simulink model "EVX_Lap_Simulation"  (R2018b)
settings: Solver=FixedStepAuto  StartTime=0  StopTime=100  FixedStep=0.01  MinStep=0.001  RelTol=1e-3
undefined symbols (not defined in the file): Car, dist, DOD, initial_velocity, motorefficiency, motormaxtorque, motorspeedradps, R0model, theta_d, Track_Dist, velocity_dnew, VoltageDOD, x, y
libraries: simulink x4
(part 2 of 3)

== system EVX_Lap_Simulation/EVX Vehicle Model/Powertrain/Brakes ==
  %_Pedal : Inport
  Constant : Constant  Value=2
  Divide : Product  Inputs=*/
  Divide1 : Product  Inputs=*/
  Front Brake Force : Gain  Gain=3000
  Rear Brake Force : Gain  Gain=1500
  Saturation : Saturate  UpperLimit=0  LowerLimit=-1000000
  Wheel Radius Rr : Gain  Gain=0.2
  Wheel radius Fr : Gain  Gain=0.2
  Rear Left Brake : Outport
  Front Left Brake : Outport  Port=2
  Front Right Brake : Outport  Port=3
  Rear Right Brake : Outport  Port=4
  tag scope: T_BrakeFront=global, T_BrakeRear=global
  wires:
  %_Pedal/1 -> Saturation/1
  Rear Brake Force/1 -> Wheel Radius Rr/1
  Front Brake Force/1 -> Wheel radius Fr/1
  Wheel Radius Rr/1 -> Divide1/1, [T_BrakeRear]
  Wheel radius Fr/1 -> Divide/1, [T_BrakeFront]
  Constant/1 -> Divide1/2, Divide/2
  Divide1/1 -> Rear Right Brake/1, Rear Left Brake/1
  Divide/1 -> Front Right Brake/1, Front Left Brake/1
  Saturation/1 -> Rear Brake Force/1, Front Brake Force/1

== system EVX_Lap_Simulation/EVX Vehicle Model/Powertrain/Motor Configuration ==
  %_Pedal : Inport
  radps_Motor1 : Inport  Port=2
  radps_Motor2 : Inport  Port=3
  radps_Motor3 : Inport  Port=4
  radps_Motor4 : Inport  Port=5
  Four Motors : Subsystem  VariantControl=FourMotor
  One Motor : Subsystem  VariantControl=OneMotor
  Two Motors : Subsystem  VariantControl=TwoMotor
  T_FL : Outport
  T_FR : Outport  Port=2
  T_RL : Outport  Port=3
  T_RR : Outport  Port=4
  P_Motor : Outport  Port=5

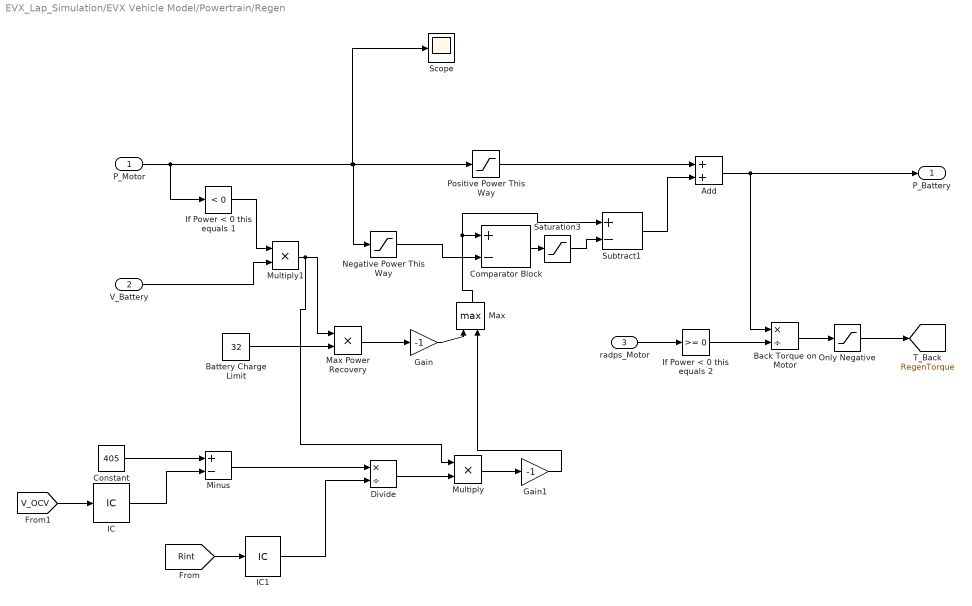
== system EVX_Lap_Simulation/EVX Vehicle Model/Powertrain/Regen ==
  P_Motor : Inport
  V_Battery : Inport  Port=2
  radps_Motor : Inport  Port=3
  Add : Sum
  Back Torque on Motor : Product  Inputs=*/
  Battery Charge Limit : Constant  Value=32
  Comparator Block : Sum  Inputs=+-
  Constant : Constant  Value=405
  Divide : Product  Inputs=*/
  Gain : Gain  Gain=-1
  Gain1 : Gain  Gain=-1
  IC : InitialCondition  Value=400
  IC1 : InitialCondition  Value=0.02
  If Power < 0 this equals 1 : simulink/Logic and Bit Operations/Compare To Zero  relop=<  OutDataTypeStr=boolean
  If Power < 0 this equals 2 : simulink/Logic and Bit Operations/Compare To Zero  relop=>=  OutDataTypeStr=boolean
  Max : MinMax  Function=max  Inputs=2
  Max Power Recovery : Product
  Minus : Sum  Inputs=+-
  Multiply : Product
  Multiply1 : Product
  Negative Power This Way : Saturate  UpperLimit=0  LowerLimit=-10000000
  Only Negative : Saturate  UpperLimit=0  LowerLimit=-10000
  Positive Power This Way : Saturate  UpperLimit=100000  LowerLimit=0
  Saturation3 : Saturate  UpperLimit=0  LowerLimit=-100000
  Scope : Scope
  Subtract1 : Sum  Inputs=+-
  P_Battery : Outport
  tag scope: RegenTorque=global
  wires:
  P_Motor/1 -> Scope/1, Negative Power This Way/1, Positive Power This Way/1, If Power < 0 this equals 1/1
  Positive Power This Way/1 -> Add/1
  Add/1 -> P_Battery/1, Back Torque on Motor/1
  V_Battery/1 -> Multiply1/2
  If Power < 0 this equals 1/1 -> Multiply1/1
  Max Power Recovery/1 -> Gain/1
  radps_Motor/1 -> If Power < 0 this equals 2/1
  Back Torque on Motor/1 -> Only Negative/1
  Only Negative/1 -> [RegenTorque]
  Battery Charge Limit/1 -> Max Power Recovery/2
  Multiply1/1 -> Multiply/1, Max Power Recovery/1
  Negative Power This Way/1 -> Comparator Block/2
  Comparator Block/1 -> Saturation3/1
  Saturation3/1 -> Subtract1/2
  Subtract1/1 -> Add/2
  Minus/1 -> Divide/1
  Constant/1 -> Minus/1
  [V_OCV] -> IC/1
  Divide/1 -> Multiply/2
  Multiply/1 -> Gain1/1
  Gain/1 -> Max/1
  Gain1/1 -> Max/2
  Max/1 -> Subtract1/1, Comparator Block/1
  IC/1 -> Minus/2
  IC1/1 -> Divide/2
  [Rint] -> IC1/1
  If Power < 0 this equals 2/1 -> Back Torque on Motor/2

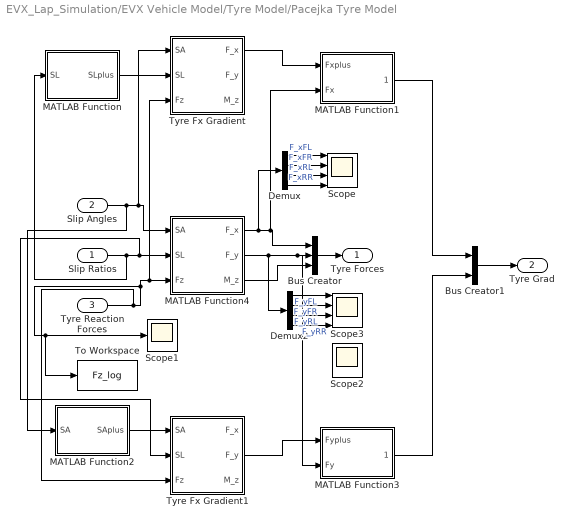
== system EVX_Lap_Simulation/EVX Vehicle Model/Tyre Model/Pacejka Tyre Model ==
  Slip Ratios : Inport
  Slip Angles : Inport  Port=2
  Tyre Reaction Forces : Inport  Port=3
  Bus Creator : BusCreator  Inputs=3
  Bus Creator1 : BusCreator  Inputs=2
  Demux : Demux
  Demux2 : Demux
  MATLAB Function : MATLAB Function  TreatAsAtomicUnit=on
  MATLAB Function1 : MATLAB Function  TreatAsAtomicUnit=on
  MATLAB Function2 : MATLAB Function  TreatAsAtomicUnit=on
  MATLAB Function3 : MATLAB Function  TreatAsAtomicUnit=on
  MATLAB Function4 : MATLAB Function  TreatAsAtomicUnit=on
  Scope : Scope  NumInputPorts=4
  Scope1 : Scope
  Scope2 : Scope  NumInputPorts=4
  Scope3 : Scope  NumInputPorts=4
  To Workspace : ToWorkspace  VariableName=Fz_log  SaveFormat=Timeseries  SampleTime=-1
  Tyre Fx Gradient : MATLAB Function  TreatAsAtomicUnit=on
  Tyre Fx Gradient1 : MATLAB Function  TreatAsAtomicUnit=on
  Tyre Forces : Outport
  Tyre Grad : Outport  Port=2
  wires:
  Bus Creator/1 -> Tyre Forces/1
  Slip Ratios/1 -> MATLAB Function/1(SL), Tyre Fx Gradient1/2(SL), MATLAB Function4/2(SL)
  Slip Angles/1 -> MATLAB Function2/1(SA), Tyre Fx Gradient/1(SA), MATLAB Function4/1(SA)
  Tyre Reaction Forces/1 -> Tyre Fx Gradient1/3(Fz), To Workspace/1, Scope1/1, Tyre Fx Gradient/3(Fz), MATLAB Function4/3(Fz)
  MATLAB Function4/1(F_x) -> Demux/1, MATLAB Function1/2(Fx), Bus Creator/1
  MATLAB Function4/2(F_y) -> Demux2/1, MATLAB Function3/2(Fy), Bus Creator/2
  MATLAB Function4/3(M_z) -> Bus Creator/3
  Demux/1 -> Scope/1  "F_xFL"
  Demux/2 -> Scope/2  "F_xFR"
  Demux/3 -> Scope/3  "F_xRL"
  Demux/4 -> Scope/4  "F_xRR"
  Demux2/1 -> Scope3/1  "F_yFL"
  Demux2/2 -> Scope3/2  "F_yFR"
  Demux2/3 -> Scope3/3  "F_yRL"
  Demux2/4 -> Scope3/4  "F_yRR"
  MATLAB Function/1(SLplus) -> Tyre Fx Gradient/2(SL)
  Tyre Fx Gradient/1(F_x) -> MATLAB Function1/1(Fxplus)
  MATLAB Function2/1(SAplus) -> Tyre Fx Gradient1/1(SA)
  Tyre Fx Gradient1/2(F_y) -> MATLAB Function3/1(Fyplus)
  MATLAB Function1/1(FxGrad) -> Bus Creator1/1
  MATLAB Function3/1(FyGrad) -> Bus Creator1/2
  Bus Creator1/1 -> Tyre Grad/1

== system EVX_Lap_Simulation/EVX Vehicle Model/Vertical Dynamics/Signal Sorting ==
  Signals : Inport
  Bus Creator : BusCreator  Inputs=8
  Bus Creator1 : BusCreator  Inputs=8
  Bus Creator2 : BusCreator  Inputs=8
  Bus Creator3 : BusCreator  Inputs=4
  Bus Creator4 : BusCreator  Inputs=4
  Bus Selector : BusSelector  OutputSignals=A,V,D,Tyre Reaction Forces
  Demux : Demux  Outputs=8
  Demux1 : Demux  Outputs=8
  Demux2 : Demux  Outputs=8
  Demux3 : Demux
  Gain{,1..8} (9 alike) : Gain  Gain=180/pi()
  Named Signals : Outport
  wires:
  Signals/1 -> Bus Selector/1
  Demux/2 -> Bus Creator/2  "Front Right (m)"
  Demux/3 -> Bus Creator/3  "Rear Left (m)"
  Demux/1 -> Bus Creator/1  "Front Left (m)"
  Demux/4 -> Bus Creator/4  "Rear Right (m)"
  Demux/5 -> Bus Creator/5  "Chassis z (m)"
  Demux/6 -> Gain/1  "Pitch (rad)"
  Demux/7 -> Gain1/1  "Front Roll (rad)"
  Demux/8 -> Gain2/1  "Rear Roll (rad)"
  Gain/1 -> Bus Creator/6  "Pitch (deg)"
  Gain2/1 -> Bus Creator/8  "Rear Roll (deg)"
  Gain1/1 -> Bus Creator/7  "Front Roll (deg)"
  Demux1/3 -> Bus Creator1/3  "Rear Left (m/s)"
  Demux1/2 -> Bus Creator1/2  "Front Right (m/s)"
  Gain4/1 -> Bus Creator1/7  "Front Roll (deg/s)"
  Gain5/1 -> Bus Creator1/8  "Rear Roll (deg/s)"
  Demux1/5 -> Bus Creator1/5  "Chassis z (m/s)"
  Demux1/6 -> Gain3/1  "Pitch (rad/s)"
  Demux1/1 -> Bus Creator1/1  "Front Left (m/s)"
  Demux1/8 -> Gain5/1  "Rear Roll (rad/s)"
  Demux1/4 -> Bus Creator1/4  "Rear Right (m/s)"
  Gain3/1 -> Bus Creator1/6  "Pitch (deg/s)"
  Demux1/7 -> Gain4/1  "Front Roll (rad/s)"
  Demux2/4 -> Bus Creator2/4  "Rear Right (m/s^2)"
  Demux2/6 -> Gain6/1  "Pitch (rad/s^2)"
  Demux2/2 -> Bus Creator2/2  "Front Right (m/s^2)"
  Demux2/8 -> Gain8/1  "Rear Roll (rad/s^2)"
  Demux2/1 -> Bus Creator2/1  "Front Left (m/s^2)"
  Demux2/5 -> Bus Creator2/5  "Chassis z (m/s^2)"
  Gain8/1 -> Bus Creator2/8  "Rear Roll (deg/s^2)"
  Gain7/1 -> Bus Creator2/7  "Front Roll (deg/s^2)"
  Demux2/7 -> Gain7/1  "Front Roll (rad/s^2)"
  Demux2/3 -> Bus Creator2/3  "Rear Left (m/s^2)"
  Gain6/1 -> Bus Creator2/6  "Pitch (deg/s^2)"
  Bus Selector/2 -> Demux1/1  "<V>"
  Bus Selector/4 -> Demux3/1  "<Tyre Reaction Forces>"
  Demux3/3 -> Bus Creator3/3  "Rear Left (N)"
  Demux3/4 -> Bus Creator3/4  "Rear Right (N)"
  Demux3/2 -> Bus Creator3/2  "Front Right (N)"
  Demux3/1 -> Bus Creator3/1  "Front Left (N)"
  Bus Creator3/1 -> Bus Creator4/4  "Tyre Forces"
  Bus Creator1/1 -> Bus Creator4/2  "Velocities"
  Bus Creator4/1 -> Named Signals/1  "Vertical Dynamics"
  Bus Selector/1 -> Demux2/1  "<A>"
  Bus Creator/1 -> Bus Creator4/3  "Displacements"
  Bus Selector/3 -> Demux/1  "<D>"
  Bus Creator2/1 -> Bus Creator4/1  "Accelerations"

== system EVX_Lap_Simulation/EVX Vehicle Model/Horizontal Dynamics/Local Dynamics/Subsystem ==
  Signals : Inport
  Bus Creator{,1..3} (4 alike) : BusCreator  Inputs=3
  Bus Selector : BusSelector  OutputSignals=Accelerations,Velocities,Displacements
  Bus Selector1 : BusSelector  OutputSignals=a_x,a_y,ddtheta_z
  Bus Selector2 : BusSelector  OutputSignals=v_x,v_y,dtheta_z
  Bus Selector3 : BusSelector  OutputSignals=d_x,d_y,theta_z
  Named Signals : Outport
  wires:
  Signals/1 -> Bus Selector/1
  Bus Selector/1 -> Bus Selector1/1  "<Accelerations>"
  Bus Selector/2 -> Bus Selector2/1  "<Velocities>"
  Bus Selector/3 -> Bus Selector3/1  "<Displacements>"
  Bus Selector1/1 -> Bus Creator/1  "<a_x>"
  Bus Selector1/2 -> Bus Creator/2  "<a_y>"
  Bus Selector1/3 -> Bus Creator/3  "<ddtheta_z>"
  Bus Selector2/1 -> Bus Creator2/1  "<v_x>"
  Bus Selector2/2 -> Bus Creator2/2  "<v_y>"
  Bus Selector2/3 -> Bus Creator2/3  "<dtheta_z>"
  Bus Selector3/2 -> Bus Creator1/2  "<d_y>"
  Bus Selector3/1 -> Bus Creator1/1  "<d_x>"
  Bus Selector3/3 -> Bus Creator1/3  "<theta_z>"
  Bus Creator2/1 -> Bus Creator3/2  "Velocities"
  Bus Creator/1 -> Bus Creator3/1  "Accelerations"
  Bus Creator1/1 -> Bus Creator3/3  "Displacements"
  Bus Creator3/1 -> Named Signals/1  "Horizontal Dynamics"

== system EVX_Lap_Simulation/EVX Vehicle Model/Powertrain/Battery/Energy ==
  P_Battery : Inport
  Battery Capacity (J) : Constant  Value=25200000
  Battery Percentage : Scope
  Divide : Product  Inputs=/*
  Energy Consumed (J) : Scope
  Energy Remaining (J) : Scope
  Gain : Gain  Gain=100
  Integrator : Integrator
  Minus : Sum  Inputs=+-
  tag scope: E_Battery=global, E_Used=global
  wires:
  Battery Capacity (J)/1 -> Divide/1, Minus/1
  Minus/1 -> Divide/2, [E_Battery], Energy Remaining (J)/1
  Integrator/1 -> Minus/2, [E_Used], Energy Consumed (J)/1
  P_Battery/1 -> Integrator/1
  Divide/1 -> Gain/1
  Gain/1 -> Battery Percentage/1

== system EVX_Lap_Simulation/EVX Vehicle Model/Powertrain/Battery/Heat Generation and Cooling ==
  I_Battery : Inport
  v_Car : Inport  Port=2
  Heat Dissipation (W) : Scope
  Heat Energy (J) : Scope
  Integrator : Integrator
  Internal Resisiatnce : Subsystem
  Multiply : Product
  Square : Math  Operator=square  SaturateOnIntegerOverflow=on
  Temperature and Cooling : Subsystem
  tag scope: E_BatteryHeat=global, P_BatteryHeat=global
  wires:
  Multiply/1 -> [P_BatteryHeat], Temperature and Cooling/1(Heat Generation), Heat Dissipation (W)/1, Integrator/1
  Square/1 -> Multiply/2
  I_Battery/1 -> Square/1
  Integrator/1 -> [E_BatteryHeat], Heat Energy (J)/1
  Internal Resisiatnce/1(R0) -> Multiply/1
  [I_cell] -> Internal Resisiatnce/2(I_cell)
  [SOC_Battery] -> Internal Resisiatnce/1(SOC_Battery)
  v_Car/1 -> Temperature and Cooling/2(v_Car)
  Temperature and Cooling/1(T_Battery) -> Internal Resisiatnce/3(T_Battery)

== system EVX_Lap_Simulation/EVX Vehicle Model/Powertrain/Battery/SOAP ==
  Vocv : Inport
  Divide : Product  Inputs=*/
  Divide2 : Product  Inputs=*/
  Multiply2 : Product
  Scope : Scope
  Subtract1 : Sum  Inputs=+-
  Vcut-off : Constant  Value=242
  tag scope: SOAP_Battery=global, SOAP_ratio=global
  wires:
  Vcut-off/1 -> Subtract1/2
  [Rint] -> Divide2/2
  Subtract1/1 -> Divide2/1
  Divide2/1 -> Multiply2/1
  [V_Battery] -> Multiply2/2
  Multiply2/1 -> Divide/1, Scope/1, [SOAP_Battery]
  Vocv/1 -> Subtract1/1
  [P_Battery] -> Divide/2
  Divide/1 -> [SOAP_ratio]

== system EVX_Lap_Simulation/EVX Vehicle Model/Powertrain/Battery/SOC ==
  Q_Battery : Inport
  %_SOC : Scope
  100% SOC : Constant  Value=72000  VectorParams1D=off
  Battery Charge (As) : Scope
  Divide1 : Product  Inputs=*/
  Gain : Gain  Gain=100
  Minus1 : Sum  Inputs=+-
  SOC_Battery : Outport
  tag scope: SOC_Battery=global
  wires:
  Gain/1 -> [SOC_Battery], SOC_Battery/1, %_SOC/1
  Divide1/1 -> Gain/1
  Minus1/1 -> Battery Charge (As)/1, Divide1/1
  100% SOC/1 -> Divide1/2, Minus1/1
  Q_Battery/1 -> Minus1/2

== system EVX_Lap_Simulation/EVX Vehicle Model/Powertrain/Battery/Voltage ==
  DOD_Battery : Inport
  Multiply1 : Product
  SOC to Voltage Look-Up Table : Lookup_n-D  NumberOfTableDimensions=1  BreakpointsForDimension1=DOD  Table=VoltageDOD  ExtrapMethod=Clip  InternalRulePriority=Speed  RndMeth=Simplest  InputSameDT=on
  Subtract : Sum  Inputs=+-
  V_Battery : Outport
  V_OCV : Outport  Port=2
  tag scope: V_OCV=global
  wires:
  Multiply1/1 -> Subtract/2
  [I_Battery] -> Multiply1/2
  [Rint] -> Multiply1/1
  DOD_Battery/1 -> SOC to Voltage Look-Up Table/1
  SOC to Voltage Look-Up Table/1 -> [V_OCV], V_OCV/1, Subtract/1
  Subtract/1 -> V_Battery/1

== system EVX_Lap_Simulation/EVX Vehicle Model/Powertrain/Motor Configuration/Four Motors ==
  " " : Inport
  %_Pedal : Inport  Port=2
  Add : Sum  Inputs=+-
  T_FL : Outport
  wires:
  %_Pedal/1 -> Add/2
  " "/1 -> Add/1
  Add/1 -> T_FL/1

== system EVX_Lap_Simulation/EVX Vehicle Model/Powertrain/Motor Configuration/One Motor ==
  %_Pedal : Inport
  radps_Motor1 : Inport  Port=2
  Add : Sum
  IC : InitialCondition
  Motor : Subsystem
  Motor Controller : Subsystem
  Multiply : Product
  Saturation : Saturate  UpperLimit=100000  LowerLimit=0
  Scope : Scope  NumInputPorts=2
  Transmission System : Subsystem
  P_Motor : Outport
  T_FL : Outport  Port=2
  T_FR : Outport  Port=3
  T_RL : Outport  Port=4
  T_RR : Outport  Port=5
  tag scope: P_Motor=global, T_Motor=global
  wires:
  Motor/1(T_Motor) -> [T_Motor], Saturation/1
  Motor Controller/1("T_Cmd ") -> Multiply/2, Motor/1(T_Cmd)
  Transmission System/2(T_FR) -> T_FR/1
  Transmission System/1(T_FL) -> T_FL/1
  Saturation/1 -> Add/1
  Multiply/1 -> [P_Motor], P_Motor/1
  radps_Motor1/1 -> Motor/2(radps_Motor1), Motor Controller/2(radps_Motor), Multiply/1
  Transmission System/3(T_RL) -> T_RL/1
  Transmission System/4(T_RR) -> T_RR/1
  Add/1 -> Transmission System/1(T_Motor)
  %_Pedal/1 -> Scope/2, Motor Controller/1(%_Pedal)
  IC/1 -> Scope/1, Add/2
  [RegenTorque] -> IC/1

== system EVX_Lap_Simulation/EVX Vehicle Model/Powertrain/Motor Configuration/Two Motors ==
  %_Pedal : Inport
  radps_Motor2 : Inport  Port=2
  radps_Motor3 : Inport  Port=3
  P_Motor : Outport
  T_FL : Outport  Port=2
  T_FR : Outport  Port=3
  T_RL : Outport  Port=4
  T_RR : Outport  Port=5

== system EVX_Lap_Simulation/EVX Vehicle Model/Powertrain/Battery/Heat Generation and Cooling/Internal Resisiatnce ==
  SOC_Battery : Inport
  I_cell : Inport  Port=2
  T_Battery : Inport  Port=3
  3-D Lookup Table : Lookup_n-D  NumberOfTableDimensions=3  BreakpointsForDimension1=[20:10:90]  BreakpointsForDimension2=[-4 -2.5 -1.25 0.5 2.5 5 10 20]  BreakpointsForDimension3=[20 40 60]  Table=R0model  InternalRulePriority=Speed  RndMeth=Simplest  InputSameDT=on
  Add : Sum
  Contact Resistance : Constant  Value=0.09
  Gain : Gain  Gain=12
  R0 : Outport
  tag scope: R_Cell=global, Rint=global
  wires:
  Add/1 -> R0/1, [Rint]
  Gain/1 -> Add/1
  3-D Lookup Table/1 -> [R_Cell], Gain/1
  Contact Resistance/1 -> Add/2
  SOC_Battery/1 -> 3-D Lookup Table/1
  I_cell/1 -> 3-D Lookup Table/2
  T_Battery/1 -> 3-D Lookup Table/3

== system EVX_Lap_Simulation/EVX Vehicle Model/Powertrain/Battery/Heat Generation and Cooling/Temperature and Cooling ==
  Heat Generation : Inport
  v_Car : Inport  Port=2
  A : Constant  Value=0.5
  Add1 : Sum
  Cp : Constant  Value=640
  Divide : Product  Inputs=*/
  Integrator1 : Integrator
  MATLAB Function : MATLAB Function  TreatAsAtomicUnit=on
  Minus : Sum  Inputs=+-
  Minus1 : Sum  Inputs=+-
  Multiply1 : Product
  Multiply2 : Product
  Multiply3 : Product
  Tamb : Constant  Value=20
  Tinit : Constant  Value=20
  Tinitial : InitialCondition  Value=20
  m : Constant  Value=34.5
  T_Battery : Outport
  tag scope: T_Battery=global
  wires:
  m/1 -> Multiply3/1
  Tinitial/1 -> Minus1/1
  Heat Generation/1 -> Minus/1
  Minus1/1 -> Multiply2/2
  v_Car/1 -> MATLAB Function/1(v_Car)
  Divide/1 -> Integrator1/1
  Multiply2/1 -> Minus/2
  Multiply3/1 -> Divide/2
  Minus/1 -> Divide/1
  MATLAB Function/1(h) -> Multiply1/1
  Integrator1/1 -> Add1/1
  Multiply1/1 -> Multiply2/1
  Tinit/1 -> Add1/2
  A/1 -> Multiply1/2
  Cp/1 -> Multiply3/2
  Tamb/1 -> Minus1/2
  Add1/1 -> [T_Battery], T_Battery/1, Tinitial/1

== system EVX_Lap_Simulation/EVX Vehicle Model/Powertrain/Motor Configuration/One Motor/Motor ==
  T_Cmd : Inport
  radps_Motor1 : Inport  Port=2
  Efficiency Map : Lookup_n-D  BreakpointsForDimension1=[-240:40:240]  BreakpointsForDimension2=[0:1000:5000]  Table=motorefficiency  InternalRulePriority=Speed  RndMeth=Simplest  InputSameDT=on
  Gain : Gain  Gain=0.01
  Multiply : Product
  T_Motor : Outport
  wires:
  T_Cmd/1 -> Multiply/1, Efficiency Map/1
  radps_Motor1/1 -> Efficiency Map/2
  Efficiency Map/1 -> Gain/1
  Multiply/1 -> T_Motor/1
  Gain/1 -> Multiply/2

== system EVX_Lap_Simulation/EVX Vehicle Model/Powertrain/Motor Configuration/One Motor/Motor Controller ==
  %_Pedal : Inport
  radps_Motor : Inport  Port=2
  Constant : Constant  Value=80000
  Divide : Product  Inputs=*/
  Divide1 : Product  Inputs=*/
  If Power < 0 this equals 2 : simulink/Logic and Bit Operations/Compare To Zero  relop=>=  OutDataTypeStr=boolean
  Max Power : Gain
  Min : MinMax  Inputs=2
  MotorMaxTorque1 : Lookup_n-D  NumberOfTableDimensions=1  BreakpointsForDimension1=motorspeedradps  Table=motormaxtorque  ExtrapMethod=Clip  InternalRulePriority=Speed  RndMeth=Simplest  InputSameDT=on
  Multiply : Product
  Saturation2 : Saturate  UpperLimit=10000  LowerLimit=0
  Subtract : Sum  Inputs=+-
  Subtract1 : Sum  Inputs=+-
  "T_Cmd " : Outport
  tag scope: radps_motor=global
  wires:
  %_Pedal/1 -> Multiply/1
  Multiply/1 -> Subtract1/1, Subtract/1
  Subtract/1 -> Saturation2/1
  Saturation2/1 -> Subtract1/2
  Subtract1/1 -> "T_Cmd "/1
  Constant/1 -> Divide/1
  [SOAP_Battery] -> Divide1/1
  radps_Motor/1 -> MotorMaxTorque1/1, [radps_motor], If Power < 0 this equals 2/1, Divide/2
  Divide/1 -> Min/1
  Divide1/1 -> Min/2
  Min/1 -> Subtract/2
  Max Power/1 -> Multiply/2
  MotorMaxTorque1/1 -> Max Power/1
  If Power < 0 this equals 2/1 -> Divide1/2

== system EVX_Lap_Simulation/EVX Vehicle Model/Powertrain/Motor Configuration/One Motor/Transmission System ==
  T_Motor : Inport
  Constant : Constant  Value=2
  Constant1 : Constant  Value=0
  Constant2 : Constant  Value=0
  Divide : Product  Inputs=*/
  Transmission Ratio : Gain  Gain=3
  T_FL : Outport
  T_FR : Outport  Port=2
  T_RL : Outport  Port=3
  T_RR : Outport  Port=4
  tag scope: T_LR=global, T_RR=global
  wires:
  Constant/1 -> Divide/2
  Transmission Ratio/1 -> Divide/1
  T_Motor/1 -> Transmission Ratio/1
  Constant1/1 -> T_FL/1
  Constant2/1 -> T_FR/1
  Divide/1 -> [T_RR], T_RR/1, [T_LR], T_RL/1

== matlab function EVX_Lap_Simulation/Limiting Factors/Traction Limit ==
  data: Pedal input; Limit output; Tyre_Grad input
function Limit = Trac_Lim(Pedal,Tyre_Grad)

Grad = (Tyre_Grad(3) + Tyre_Grad(4))/2;

if Pedal > 0 && Grad <= 0
    Limit = 1;
else
    Limit = 0;
end

== matlab function EVX_Lap_Simulation/Limiting Factors/Power Limit ==
  data: Pedal input; Limit output
function Limit = Pedal_Lim(Pedal)

if Pedal == 100
    Limit = 1;
else 
    Limit = 0;
end

== matlab function EVX_Lap_Simulation/Limiting Factors/Braking Limit ==
  data: Pedal input; Limit output; Tyre_Grad input
function Limit = Brake_Lim(Pedal,Tyre_Grad)

Grad = (sum(Tyre_Grad))/4;

if Pedal < 0 && Grad <= 0
    Limit = 1;
elseif Pedal == -100
    Limit = 1;
else
    Limit = 0;
end

== matlab function EVX_Lap_Simulation/Limiting Factors/Cornering Limit ==
  data: Tyre_Grad input; Limit output
function Limit = Corner_Lim(Tyre_Grad)

Grad = (Tyre_Grad(1) + Tyre_Grad(2))/2;

if Grad <= 0
    Limit = 1;
else
    Limit = 0;
end

== matlab function EVX_Lap_Simulation/Limiting Factors/MATLAB Function ==
  data: Power_Lim input; Limit output; Trac_Lim input; Brake_Lim input; Corner_Lim input
function Limit = Overall_Lim(Power_Lim,Trac_Lim,Brake_Lim,Corner_Lim)

Limit = max([Power_Lim,Trac_Lim,Brake_Lim,Corner_Lim]);

== matlab function EVX_Lap_Simulation/EVX Vehicle Model/Powertrain/Battery/Heat Generation and Cooling/Temperature and Cooling/MATLAB Function ==
  data: v_Car input; h output
function h = fcn(v_Car)

h = 10.45-v_Car+10*sqrt(max(v_Car,0));

== matlab function EVX_Lap_Simulation/EVX Vehicle Model/Powertrain/Reverse Transmission Function1 ==
  data: Ratio input; data input; Motor_Speed output; dwheel input
function Motor_Speed = Rev_Transmission(Ratio,data, dwheel)

Motor_Speed = ((dwheel(3) + dwheel(4)) / 2) * Ratio;

== matlab function EVX_Lap_Simulation/EVX Vehicle Model/Powertrain/MATLAB Function ==
  data: pedal input; out output
function out = fcn(pedal)

out = [0;0;240;240].*pedal./100;

== matlab function EVX_Lap_Simulation/Driver Model/Control System Driver Model/MATLAB Function ==
  data: u input; v input; a_req output; t input
function a_req = fcn(u,v,t)

a_req = (v - u)/t;

== matlab function EVX_Lap_Simulation/Stopping Criteria/MATLAB Function8 ==
  data: x input; Stop output; y input; dist_cur input; dist_end input; t input
function Stop = LapEnd(x,y,dist_cur,dist_end,t)

if abs(x) < 1 && y <=1 && t > 10
    Stop = 1;
elseif dist_cur >= dist_end
    Stop = 1;
else
    Stop = 0;
end

== matlab function EVX_Lap_Simulation/EVX Vehicle Model/Aero Model/Forces ==
  data: v_x input; F_L output; F_D output
function [F_L,F_D] = fcn(v_x)

rho = 1.19;
A = 1.5*1.5; % Frontal area (dependant on ride height) RANDOM - NEEDS UPDATING
C_L = 1; % Coefficient of lift RANDOM - NEEDS UPDATING
C_D = 0.5; % Coefficient of drag RANDOM - NEEDS UPDATING

F_L = 0.5*rho*(v_x^2)*A*C_L;
F_D = 0.5*rho*(v_x^2)*A*C_D;

== matlab function EVX_Lap_Simulation/EVX Vehicle Model/Aero Model/Position ==
  data: v_x input; L output; D output
function [L,D] = fcn(v_x)

L_x = 0.8;
L_y = 0.0;
L_z = 0.5;

D_x = 0.5;
D_y = 0;
D_z = 0.4;

L = [L_x,L_y,L_z];

D = [D_x,D_y,D_z];

== matlab function EVX_Lap_Simulation/EVX Vehicle Model/Horizontal Dynamics/Acceleration Forces ==
  data: a_x input; a_y input; ddtheta_z input; m input; h input; w input; M_y output; M_xF output; M_xR output
function [M_y,M_xF,M_xR] = fcn(a_x,a_y,ddtheta_z,m,h,w)

M_y = -m(5) * a_x * h(1);

a_yF = a_y + w(1,1)/2 * ddtheta_z;
a_yR = a_y + w(1,3)/2 * ddtheta_z;

M_xF = m(6) * a_yF * h(2);
M_xR = m(7) * a_yR * h(3);

== matlab function EVX_Lap_Simulation/EVX Vehicle Model/Horizontal Dynamics/Aero_Forces ==
  data: F_L input; F_D input; F_x output; l input; d input; F_zC output; M_x output; M_y output; M_z output
function [F_x,F_zC,M_x,M_y,M_z] = Aero_Forces(F_L,F_D,l,d)

F_zC = -F_L;
M_x = F_L * l(2);
M_y = F_L * l(1);

F_x = -F_D;
M_y = M_y + -F_D * d(3);
M_z = F_D * d(2);

== matlab function EVX_Lap_Simulation/EVX Vehicle Model/Horizontal Dynamics/F=ma ==
  data: F_x input; a_x output; F_y input; M_z input; m input; I input; a_y output; ddtheta_z output
function [a_x,a_y,ddtheta_z] = F_ma(F_x,F_y,M_z,m,I)

mass = m(1) + m(2) + m(3) + m(4) + m(5);

a_x = F_x / mass;
a_y = F_y / mass;
ddtheta_z = M_z / I(4);

== matlab function EVX_Lap_Simulation/EVX Vehicle Model/Horizontal Dynamics/Gravitational_Forces ==
  data: m input; F_zFL output; g input; F_zFR output; F_zRL output; F_zRR output; F_zC output
function [F_zFL,F_zFR,F_zRL,F_zRR,F_zC] = Grav_Forces(m,g)

F_zFL = g * m(1);
F_zFR = g * m(2);
F_zRL = g * m(3);
F_zRR = g * m(4);
F_zC = g * m(5);

% F = [F_zFL,F_zFR,F_zRL,F_zRR,F_zC];

== matlab function EVX_Lap_Simulation/EVX Vehicle Model/Horizontal Dynamics/MATLAB Function ==
  data: M_x input; M_xF output; M_xR output
function [M_xF,M_xR] = fcn(M_x)

M_xF = 0.5 * M_x;
M_xR = 0.5 * M_x;

== matlab function EVX_Lap_Simulation/EVX Vehicle Model/Horizontal Dynamics/Position Conversion ==
  data: L input; l output; D input; w input; d output; h input
function [l,d] = fcn(L,D,w,h)

l_x = w(1) - L(1);
l_y = L(2)-((w(2,1) - w(2,2))/2 - w(2,1));
l_z = L(3) - h(1);

l = [l_x,l_y,l_z];

d_x = w(1) - D(1);
d_y = D(2)-((w(2,1) - w(2,2))/2 - w(2,1));
d_z = D(3) - h(1);

d = [d_x,d_y,d_z];

== matlab function EVX_Lap_Simulation/EVX Vehicle Model/Horizontal Dynamics/Tyre_Forces ==
  data: F_TxFL input; F_x output; F_TxFR input; F_TxRL input; F_TxRR input; F_TyFL input; F_TyFR input; F_TyRL input; F_TyRR input; M_TzFL input; M_TzFR input; M_TzRL input; M_TzRR input; S input; w input; F_y output; M_z output
function [F_x,F_y,M_z] = Tyre_Forces(F_TxFL,F_TxFR,F_TxRL,F_TxRR...
    ,F_TyFL,F_TyFR,F_TyRL,F_TyRR,M_TzFL,M_TzFR,M_TzRL,M_TzRR,S,w)

F_TyRL = -F_TyRL;
F_TyRR = -F_TyRR;

F_x = zeros(1);
F_y = zeros(1);
M_z = zeros(1);

F_x = F_TxFL * cosd(S(1)) - F_TyFL * sind(S(1))...
    + F_TxFR * cosd(S(2)) - F_TyFR * sind(S(2))...
    + F_TxRL * cosd(S(3)) - F_TyRL * sind(S(3))...
    + F_TxRR * cosd(S(4)) - F_TyRR * sind(S(4));

F_y = F_TxFL * sind(S(1)) + F_TyFL * cosd(S(1))...
    + F_TxFR * sind(S(2)) + F_TyFR * cosd(S(2))...
    - F_TxRL * sind(S(3)) - F_TyRL * cosd(S(3))...
    - F_TxRR * sind(S(4)) - F_TyRR * cosd(S(4));

M_z = F_TxFL * (w(1,1) * sind(S(1)) - w(2,1) * cosd(S(1)))...
    + F_TyFL * (w(2,1) * sind(S(1)) + w(1,1) * cosd(S(1)))...
    + F_TxFR * (w(1,2) * sind(S(2)) - w(2,2) * cosd(S(2)))...
    + F_TyFR * (w(2,2) * sind(S(2)) + w(1,2) * cosd(S(2)))...
    + F_TxRL * (-w(1,3) * sind(S(3)) - w(2,3) * cosd(S(3)))...
    + F_TyRL * (w(2,3) * sind(S(3)) - w(1,3) * cosd(S(3)))...
    + F_TxRR * (-w(1,4) * sind(S(4)) - w(2,4) * cosd(S(4)))...
    + F_TyRR * (w(2,4) * sind(S(4)) - w(1,4) * cosd(S(4)))...
    - M_TzFL - M_TzFR + M_TzRL + M_TzRR;

== matlab function EVX_Lap_Simulation/Driver Model/Control System Driver Model/MATLAB Function1 ==
  data: t_grad input; a_cur input; pedal_out output; a_req input; pedal_in input
function pedal_out = fcn(t_grad,a_cur,a_req,pedal_in)

% pedal_in = 0;

if abs(a_req - a_cur) > 0.001
    pedal_out = (a_req - a_cur) * 0;
else
    pedal_out = pedal_in;
end

if t_grad < 0
    if a_cur < 0
        if a_req < a_cur
            pedal_out = 0;
        end
    elseif a_cur > 0
        if a_req > a_cur
            pedal_out = 0;
        end
    else
        pedal_out = 0;
    end
end



pedal_out(pedal_out > 100) = 100;
pedal_out(pedal_out < -100) = -100;

== matlab function EVX_Lap_Simulation/Driver Model/Control System Driver Model/MATLAB Function2 ==
  data: Fx_Grad_RL input; Fx_Grad_RR input; y output; t input
function y = fcn(Fx_Grad_RL,Fx_Grad_RR,t)

x = (Fx_Grad_RL + Fx_Grad_RR)/2;

if t < 0.001
    y = 1;
else
    y = x;
end

== matlab function EVX_Lap_Simulation/EVX Vehicle Model/Powertrain/Brake Function ==
  data: v_wx input; Pedal input; Torque output
function Torque = fcn(v_wx,Pedal)

max_T = [800;800;600;600];

Torque = max_T .* Pedal/100 .* sign(v_wx);

== matlab function EVX_Lap_Simulation/EVX Vehicle Model/Powertrain/Motor Fucntion ==
  data: Pedal input; Torque output; Motor_Speed input; Direction input
function Torque  = Motor(Pedal,Motor_Speed,Direction)

if Pedal > 100
    Pedal = 100;
elseif Pedal < 0
    Pedal = 0;
end

power = 80000;

max_torque = 240;

torque_line = abs(power / Motor_Speed) * Direction;

Torque = min(max_torque,torque_line) * (Pedal / 100);

== matlab function EVX_Lap_Simulation/EVX Vehicle Model/Powertrain/Reverse Transmission Function ==
  data: Ratio input; data input; Motor_Speed output; dwheel input
function Motor_Speed = Rev_Transmission(Ratio,data, dwheel)

Motor_Speed = ((dwheel(3) + dwheel(4)) / 2) * Ratio;

== matlab function EVX_Lap_Simulation/EVX Vehicle Model/Powertrain/Transmission Function ==
  data: T_FL output; Ratio input; T_FR output; T_RL output; Motor_Torque input; Splits input; T_RR output
function [T_FL,T_FR,T_RL,T_RR] = Transmission(Ratio,Motor_Torque,Splits)

T_FR = 0;
T_FL = T_FR;
T_RR = (Motor_Torque * Ratio) / (Splits + 1);
T_RL = T_RR;

== matlab function EVX_Lap_Simulation/EVX Vehicle Model/Steering/Front//Rear Split ==
  data: Angle input; Steering_F output; Steering_R output
function [Steering_F,Steering_R] = Steering_Split(Angle)

Steering_F = Angle;
Steering_R = 0;

== matlab function EVX_Lap_Simulation/EVX Vehicle Model/Steering/MATLAB Function ==
  data: S_FL output; Steering_F input; S_FR output; Ratio input
function [S_FL,S_FR] = Steeting_Front(Steering_F,Ratio)

S_FL = Steering_F / Ratio;
S_FR = Steering_F / Ratio;
% 
% if abs(Steering_F) > Ratio/2
%     S_FL = S_FL + 0.5;
%     S_FR = S_FR - 0.5;
% end
%

== matlab function EVX_Lap_Simulation/Driver Model/Control System Driver Model/MATLAB Function3 ==
  data: t_grad input; pedal_out output; v_cur input; v_req input; pedal_in input
function pedal_out = fcn(t_grad,v_cur,v_req,pedal_in)

if t_grad > 0
pedal_out = pedal_in + (v_req - v_cur) * 100;
else
% pedal_out = pedal_in;
pedal_out = pedal_in + (v_req - v_cur) * 100;
end

pedal_out(pedal_out > 100) = 100;
pedal_out(pedal_out < -100) = -100;

== matlab function EVX_Lap_Simulation/Driver Model/Control System Driver Model/MATLAB Function4 ==
  data: theta_req input; Steering output; theta_cur input; tyre_grad input
function Steering = fcn(theta_req,theta_cur,tyre_grad)

if tyre_grad > 0
Steering = (theta_req - theta_cur) * 250;
else
% Steering = (abs(steering_in) - 1) .* sign(steering_in);
Steering = (theta_req - theta_cur) * 125;
end

Steering(Steering > 90) = 90;
Steering(Steering < -90) = -90;

== matlab function EVX_Lap_Simulation/Driver Model/Control System Driver Model/MATLAB Function5 ==
  data: Fy_Grad_FL input; Fy_Grad_FR input; y output; t input
function y = fcn(Fy_Grad_FL,Fy_Grad_FR,t)

x = (Fy_Grad_FL + Fy_Grad_FR)/2;

if t < 0.001
    y = 1;
else
    y = x;
end

== matlab function EVX_Lap_Simulation/Driver Model/Control System Driver Model/MATLAB Function6 ==
  data: x_tar input; theta_error output; y_tar input; x_cur input; y_cur input; theta_cur input
function theta_error = Path_Cor(x_tar,y_tar,x_cur,y_cur,theta_cur)

theta_error = atan2((y_tar - y_cur),(x_tar - x_cur));

while theta_error > 1.9 * pi
    theta_error = theta_error - 2 * pi;
end

while theta_error < -1.9 * pi
    theta_error = theta_error + 2 * pi;
end

== matlab function EVX_Lap_Simulation/Driver Model/Control System Driver Model/MATLAB Function7 ==
  data: steering_in input; steering output; correction input; Tyre_grad input
function steering = fcn(steering_in,correction,Tyre_grad)

if Tyre_grad > 0
    
    steering = steering_in + correction*0;
    
else
    steering = steering_in;
    
end

== matlab function EVX_Lap_Simulation/EVX Vehicle Model/Steering/MATLAB Function1 ==
  data: S_RL output; Steering_R input; S_RR output; Ratio input
function [S_RL,S_RR] = Steeting_Rear(Steering_R,Ratio)

S_RL = Steering_R / Ratio;
S_RR = Steering_R / Ratio;

== matlab function EVX_Lap_Simulation/Driver Model/Control System Driver Model/MATLAB Function8 ==
  data: x input; dist_out output; y input; dist input; x_log input; y_log input
function dist_out = fcn(x,y,dist,x_log,y_log)

distances = ((x-x_log).^2+(y-y_log).^2).^0.5;
[~,row] = min(distances);
dist_out = dist(row);

== matlab function EVX_Lap_Simulation/Driver Model/Control System Driver Model/Next Distance1 ==
  data: Dist input; Next_Distance output; Velocity input; Acceleration input; Time_Step input
function Next_Distance = NextDist(Dist,Velocity,Acceleration,Time_Step)

Next_Distance = Dist + Velocity * Time_Step + 0.5 * Acceleration * (Time_Step)^2;

== matlab function EVX_Lap_Simulation/Driver Model1/Control System Driver Model/MATLAB Function ==
  data: u input; v input; a_req output; t input
function a_req = fcn(u,v,t)

a_req = (v - u)/t;

== matlab function EVX_Lap_Simulation/Driver Model1/Control System Driver Model/MATLAB Function1 ==
  data: t_grad input; a_cur input; pedal_out output; a_req input; pedal_in input
function pedal_out = fcn(t_grad,a_cur,a_req,pedal_in)

% pedal_in = 0;

if abs(a_req - a_cur) > 0.001
    pedal_out = (a_req - a_cur) * 0;
else
    pedal_out = pedal_in;
end

if t_grad < 0
    if a_cur < 0
        if a_req < a_cur
            pedal_out = 0;
        end
    elseif a_cur > 0
        if a_req > a_cur
            pedal_out = 0;
        end
    else
        pedal_out = 0;
    end
end



pedal_out(pedal_out > 100) = 100;
pedal_out(pedal_out < -100) = -100;

== matlab function EVX_Lap_Simulation/Driver Model1/Control System Driver Model/MATLAB Function2 ==
  data: Fx_Grad_RL input; Fx_Grad_RR input; y output; t input
function y = fcn(Fx_Grad_RL,Fx_Grad_RR,t)

x = (Fx_Grad_RL + Fx_Grad_RR)/2;

if t < 0.001
    y = 1;
else
    y = x;
end

== matlab function EVX_Lap_Simulation/Driver Model1/Control System Driver Model/MATLAB Function3 ==
  data: t_grad input; pedal_out output; v_cur input; v_req input; pedal_in input
function pedal_out = fcn(t_grad,v_cur,v_req,pedal_in)

if t_grad > 0
pedal_out = pedal_in + (v_req - v_cur) * 100;
else
% pedal_out = pedal_in;
pedal_out = pedal_in + (v_req - v_cur) * 0;
end

pedal_out(pedal_out > 100) = 100;
pedal_out(pedal_out < -100) = -100;

== matlab function EVX_Lap_Simulation/Driver Model1/Control System Driver Model/MATLAB Function4 ==
  data: theta_req input; Steering output; theta_cur input; tyre_grad input
function Steering = fcn(theta_req,theta_cur,tyre_grad)

if tyre_grad > 0
Steering = (theta_req - theta_cur) * 250;
else
% Steering = (abs(steering_in) - 1) .* sign(steering_in);
Steering = (theta_req - theta_cur) * 125;
end

Steering(Steering > 90) = 90;
Steering(Steering < -90) = -90;

== matlab function EVX_Lap_Simulation/Driver Model1/Control System Driver Model/MATLAB Function5 ==
  data: Fy_Grad_FL input; Fy_Grad_FR input; y output; t input
function y = fcn(Fy_Grad_FL,Fy_Grad_FR,t)

x = (Fy_Grad_FL + Fy_Grad_FR)/2;

if t < 0.001
    y = 1;
else
    y = x;
end

== matlab function EVX_Lap_Simulation/Driver Model1/Control System Driver Model/MATLAB Function6 ==
  data: x_tar input; theta_error output; y_tar input; x_cur input; y_cur input; theta_cur input
function theta_error = Path_Cor(x_tar,y_tar,x_cur,y_cur,theta_cur)

theta_error = atan2((y_tar - y_cur),(x_tar - x_cur));

while theta_error > 1.9 * pi
    theta_error = theta_error - 2 * pi;
end

while theta_error < -1.9 * pi
    theta_error = theta_error + 2 * pi;
end

== matlab function EVX_Lap_Simulation/Driver Model1/Control System Driver Model/MATLAB Function7 ==
  data: steering_in input; steering output; correction input; Tyre_grad input
function steering = fcn(steering_in,correction,Tyre_grad)

if Tyre_grad > 0
    
    steering = steering_in + correction*0;
    
else
    steering = steering_in;
    
end

== matlab function EVX_Lap_Simulation/Driver Model1/Control System Driver Model/MATLAB Function8 ==
  data: x input; dist_out output; y input; dist input; x_log input; y_log input
function dist_out = fcn(x,y,dist,x_log,y_log)

y = u;

== matlab function EVX_Lap_Simulation/Driver Model1/Control System Driver Model/Next Distance1 ==
  data: Dist input; Next_Distance output; Velocity input; Acceleration input; Time_Step input
function Next_Distance = NextDist(Dist,Velocity,Acceleration,Time_Step)

Next_Distance = Dist + Velocity * Time_Step + 0.5 * Acceleration * (Time_Step)^2;

== matlab function EVX_Lap_Simulation/EVX Vehicle Model/Subsystem/Car Parameters ==
  data: w output; m output; I output; kc output; cc output; h output
function [w,m,I,kc,cc,h] = Car_Param()

% Wheel Positions
a = 0.775;
b = 0.775;
d_F = 0.6;
e_F = 0.6;
d_R = 0.6;
e_R = 0.6;

w = [a,a,-b,-b;d_F,-e_F,d_R,-e_R];

% Mass & Intertias
m_WFL = 10;
m_WFR = 10;
m_WRL = 10;
m_WRR = 10;
m_c = 250;
m_cF = 125;
m_cR = m_c - m_cF;
I_cy = 50;
I_xF = 20;
I_xR = 20;
I_z = 50;

m = [m_WFL;m_WFR;m_WRL;m_WRR;m_c;m_cF;m_cR];
I = [I_cy;I_xF;I_xR;I_z];

% Chassis Stiffness
kc_x = 5000;

kc = [kc_x];

% Chassis Damping
cc_x = 500;

cc = [cc_x];

% Chassis COG Height
h_c = 0.05;
h_cF = 0.05;
h_cR = 0.05;

h = [h_c;h_cF;h_cR];

== matlab function EVX_Lap_Simulation/EVX Vehicle Model/Subsystem/Environment Parameters ==
  data: g output
function g  = Env_Param

g = -9.81;

== matlab function EVX_Lap_Simulation/EVX Vehicle Model/Subsystem/Suspension Parameters ==
  data: kt output; ks output; kr output; ct output; cs output; cr output
function [kt,ks,kr,ct,cs,cr] = Sus_Param()

% Tyre Stiffness
kt_FL = 50000;
kt_FR = 50000;
kt_RL = 50000;
kt_RR = 50000;

kt = [kt_FL;kt_FR;kt_RL;kt_RR];

% Suspension Stiffness
ks_FL = 75000;
ks_FR = 75000;
ks_RL = 75000;
ks_RR = 75000;

ks = [ks_FL;ks_FR;ks_RL;ks_RR];

% Rollbar Stiffness
kr_Fx = 0;
kr_Rx = 0;
kr_Ly = 0;
kr_Ry = 0;
kr_FLRR = 0;
kr_FRRL = 0;

kr = [kr_Fx;kr_Rx;kr_Ly;kr_Ry;kr_FLRR;kr_FRRL];

% Tyre Damping
ct_FL = 250;
ct_FR = 250;
ct_RL = 250;
ct_RR = 250;

ct = [ct_FL;ct_FR;ct_RL;ct_RR];

% Suspension Damping
cs_FL = 250;
cs_FR = 250;
cs_RL = 250;
cs_RR = 250;

cs = [cs_FL;cs_FR;cs_RL;cs_RR];

% Rollbar Damping
cr_Fx = 0;
cr_Rx = 0;
cr_Ly = 0;
cr_Ry = 0;
cr_FLRR = 0;
cr_FRRL = 0;

cr = [cr_Fx;cr_Rx;cr_Ly;cr_Ry;cr_FLRR;cr_FRRL];

== matlab function EVX_Lap_Simulation/EVX Vehicle Model/Subsystem/Wheel Parameters ==
  data: r output; I output
function [r,I] = fcn()

r_FL = 0.175;
r_FR = 0.175;
r_RL = 0.175;
r_RR = 0.175;

I_FL = 2;
I_FR = 2;
I_RL = 2;
I_RR = 2;

r = [r_FL;r_FR;r_RL;r_RR];
I = [I_FL;I_FR;I_RL;I_RR];

== matlab function EVX_Lap_Simulation/EVX Vehicle Model/Tyre Model/MATLAB Function ==
  data: r input; F_x output; T input; F_x input
function F_x = Power_Lim(r,T,F_x)

max_F = T ./ r;

if T > 0
    for i = 1:4
        F_x(i) = min(F_x(i),max_F(i));
    end
end

if T < 0
    for i = 1:4
        F_x(i) = max(F_x(i),max_F(i));
    end
end

== matlab function EVX_Lap_Simulation/EVX Vehicle Model/Tyre Model/Pacejka Tyre Model/MATLAB Function ==
  data: SL input; SLplus output
function SLplus = Add(SL)

SLplus = SL + 0.01;

== matlab function EVX_Lap_Simulation/EVX Vehicle Model/Tyre Model/Pacejka Tyre Model/MATLAB Function1 ==
  data: Fxplus input; FxGrad output; Fx input
function FxGrad = xGrad(Fxplus,Fx)

FxGrad = zeros(4,1);
FxGrad = (Fxplus - Fx) ./ 0.01;

== matlab function EVX_Lap_Simulation/EVX Vehicle Model/Tyre Model/Pacejka Tyre Model/MATLAB Function2 ==
  data: SA input; SAplus output
function SAplus = Add(SA)

SAplus = SA + 0.01;

== matlab function EVX_Lap_Simulation/EVX Vehicle Model/Tyre Model/Pacejka Tyre Model/MATLAB Function3 ==
  data: Fyplus input; FyGrad output; Fy input
function FyGrad = yGrad(Fyplus,Fy)

FyGrad = zeros(4,1);
FyGrad = (Fyplus - Fy)./ 0.01;

== matlab function EVX_Lap_Simulation/EVX Vehicle Model/Tyre Model/Pacejka Tyre Model/MATLAB Function4 ==
  data: F_x output; SA input; F_y output; SL input; Fz input; M_z output
function [F_x,F_y,M_z] = Pacejka4(SA,SL,Fz)
SL = SL .* 30;
SM = sqrt(SA.^2 + SL.^2);
B = 18.6206;
C = 0.0180;
D = 3.5223e+04.*(-Fz./180).*0.6;
E = 1.1095;
F = zeros(length(D),1);
for i = 1:length(D)
D2 = D(i);
Sv = 0; %Vertical shift
Sh = 0; %Horizontal shift

x = 0.0174533.*SM(i) + Sh;
y = D2*sin(C*atan(B*x - E*(B*x - atan(B*x))));
F(i) = y + Sv;
end
theta = atand(SL./SA);
F_x = abs(F.*sind(theta)).*sign(SL);
F_y = abs(F.*cosd(theta)).*sign(SA);
M_z = zeros(4,1);
F_x(isnan(F_x)) = 0;
F_y(isnan(F_y)) = 0;
% M_z(isnan(M_z)) = 0;
end

== matlab function EVX_Lap_Simulation/EVX Vehicle Model/Tyre Model/Pacejka Tyre Model/Tyre Fx Gradient ==
  data: F_x output; SA input; F_y output; SL input; Fz input; M_z output
function [F_x,F_y,M_z] = Pacejka4(SA,SL,Fz)
SL = SL .* 30;
SM = sqrt(SA.^2 + SL.^2);
B = 18.6206;
C = 0.0180;
D = 3.5223e+04.*(-Fz./180).*0.6;
E = 1.1095;
F = zeros(length(D),1);
for i = 1:length(D)
D2 = D(i);
Sv = 0; %Vertical shift
Sh = 0; %Horizontal shift

x = 0.0174533.*SM(i) + Sh;
y = D2*sin(C*atan(B*x - E*(B*x - atan(B*x))));
F(i) = y + Sv;
end
theta = atand(SL./SA);
F_x = abs(F.*sind(theta)).*sign(SL);
F_y = abs(F.*cosd(theta)).*sign(SA);
M_z = zeros(4,1);
F_x(isnan(F_x)) = 0;
F_y(isnan(F_y)) = 0;
M_z(isnan(M_z)) = 0;
end

== matlab function EVX_Lap_Simulation/EVX Vehicle Model/Tyre Model/Pacejka Tyre Model/Tyre Fx Gradient1 ==
  data: F_x output; SA input; F_y output; SL input; Fz input; M_z output
function [F_x,F_y,M_z] = Pacejka4(SA,SL,Fz)
SL = SL .* 30;
SM = sqrt(SA.^2 + SL.^2);
B = 18.6206;
C = 0.0180;
D = 3.5223e+04.*(-Fz./180).*0.6;
E = 1.1095;
F = zeros(length(D),1);
for i = 1:length(D)
D2 = D(i);
Sv = 0; %Vertical shift
Sh = 0; %Horizontal shift

x = 0.0174533.*SM(i) + Sh;
y = D2*sin(C*atan(B*x - E*(B*x - atan(B*x))));
F(i) = y + Sv;
end
theta = atand(SL./SA);
F_x = abs(F.*sind(theta)).*sign(SL);
F_y = abs(F.*cosd(theta)).*sign(SA);
M_z = zeros(4,1);
F_x(isnan(F_x)) = 0;
F_y(isnan(F_y)) = 0;
M_z(isnan(M_z)) = 0;
end

== matlab function EVX_Lap_Simulation/EVX Vehicle Model/Tyre Model/Slip Angle ==
  data: v_xw input; v_yw input; SA output; S input
function SA  = Slip_Angle(v_xw,v_yw,S)

% v_xw(v_xw == 0) = 0.001;

alpha = atand(v_yw ./ v_xw);

SA = S - alpha;

SA(v_yw == 0 & v_xw == 0) = 0;
SA(SA > 30) = 30;
SA(SA < -30) = -30;

== matlab function EVX_Lap_Simulation/EVX Vehicle Model/Tyre Model/Slip Ratio ==
  data: r input; dwheel input; v_xw input; SL output
function SL  = Slip_Ratio(r,dwheel,v_xw)

% v_xw(v_xw == 0) = 0.001;

SL = (((dwheel .* r) - v_xw) ./ abs(v_xw));

%limits on SL
SL(dwheel == 0 & v_xw == 0) = 0;
SL(dwheel > 0 & v_xw == 0) = 1;
SL(dwheel < 0 & v_xw == 0) = -1;
SL(SL > 1) = 1;
SL(SL < -1) = -1;

== matlab function EVX_Lap_Simulation/EVX Vehicle Model/Tyre Model/Wheel Horizontal Velocities ==
  data: v_x input; v_y input; v_xw output; dtheta_z input; w input; v_yw output
function [v_xw,v_yw] = Wheel_Velocities(v_x,v_y,dtheta_z,w)

% Wheel velocities in x direction
v_xFL = v_x - dtheta_z * w(2,1);
v_xFR = v_x - dtheta_z * w(2,2);
v_xRL = v_x - dtheta_z * w(2,3);
v_xRR = v_x - dtheta_z * w(2,4);

% Wheel velocities in y direction
v_yFL = v_y + dtheta_z * w(1,1);
v_yFR = v_y + dtheta_z * w(1,2);
v_yRL = v_y + dtheta_z * w(1,3);
v_yRR = v_y + dtheta_z * w(1,4);

v_xw = [v_xFL;v_xFR;v_xRL;v_xRR];
v_yw = [v_yFL;v_yFR;v_yRL;v_yRR];

== matlab function EVX_Lap_Simulation/EVX Vehicle Model/Vertical Dynamics/8DOF Vibrations ==
  data: V input; A output; V output; D input; F input; zB input; dzB input; D output; w input; m input; I input; kc input; cc input; kt input; ks input; kr input; ct input; cs input; cr input; kt output; ct output
function [A,V,D,kt,ct] =   DOF_Dynamics(V,D,F,zB,dzB,w,m,I,kc,cc,kt,ks,kr,ct,cs,cr)

% Tyre Stifness = 0 when off ground
for i = 1:4
    if D(i) - zB(i) > 0
        kt(i) = 0;
        ct(i) = 0;
    end
end

% Wheel Positions
x_wFL = w(1,1);
x_wFR = w(1,2);
x_wRL = w(1,3);
x_wRR = w(1,4);

y_wFL = w(2,1);
y_wFR = w(2,2);
y_wRL = w(2,3);
y_wRR = w(2,4);

% Chassis Forces
Fw_FL = F(1);
Fw_FR = F(2);
Fw_RL = F(3);
Fw_RR = F(4);
Fc_z = F(5);
Mc_y = F(6);
McF_x = F(7);
McR_x = F(8);

% Mass & Intertias
m_WFL = m(1);
m_WFR = m(2);
m_WRL = m(3);
m_WRR = m(4);
m_c = m(5);
I_cy = I(1);
I_xF = I(2);
I_xR = I(3);
I_z = I(4);

% Base Displacements
zB_FL = zB(1);
zB_FR = zB(2);
zB_RL = zB(3);
zB_RR = zB(4);

% Base Velocities
dzB_FL = dzB(1);
dzB_FR = dzB(2);
dzB_RL = dzB(3);
dzB_RR = dzB(4);

% Tyre Stiffness
kt_FL = kt(1);
kt_FR = kt(2);
kt_RL = kt(3);
kt_RR = kt(4);

% Suspension Stiffness
ks_FL = ks(1);
ks_FR = ks(2);
ks_RL = ks(3);
ks_RR = ks(4);

% Rollbar Stiffness
kr_Fx = kr(1);
kr_Rx = kr(2);
kr_Ly = kr(3);
kr_Ry = kr(4);
kr_FLRR = kr(5);
kr_FRRL = kr(6);

% Chassis Stiffness
kc_x = kc(1);

% Tyre Damping
ct_FL = ct(1);
ct_FR = ct(2);
ct_RL = ct(3);
ct_RR = ct(4);

% Suspension Damping
cs_FL = cs(1);
cs_FR = cs(2);
cs_RL = cs(3);
cs_RR = cs(4);

% Rollbar Damping
cr_Fx = cr(1);
cr_Rx = cr(2);
cr_Ly = cr(3);
cr_Ry = cr(4);
cr_FLRR = cr(5);
cr_FRRL = cr(6);

% Chassis Damping
cc_x = cc(1);

% Displacements
z_wFL = D(1);
z_wFR = D(2);
z_wRL = D(3);
z_wRR = D(4);
z_c = D(5);
thetay_c = D(6);
thetax_F = D(7);
thetax_R = D(8);

% Velocities
dz_wFL = V(1);
dz_wFR = V(2);
dz_wRL = V(3);
dz_wRR = V(4);
dz_c = V(5);
dthetay_c = V(6);
dthetax_F = V(7);
dthetax_R = V(8);

% Accelerations

ddz_wFL = (1 / m(1)) * (F(1)...
    + kt(1) * (zB(1) - D(1))...
    - ks(1) * (D(1) - D(5) + w(1,1) * D(6) - w(2,1) * D(7))...
    + ct(1) * (dzB(1) - V(1))...
    - cs(1) * (V(1) - V(5) + w(1,1) * V(6) - w(2,1) * V(7))...
    + kr(1) * (D(2) - D(1))...
    - kr(3) * (D(1) - D(3))...
    - kr(5) * (D(1) - D(4))...
    + cr(1) * (V(2) - V(1))...
    - cr(3) * (V(1) - V(3))...
    - cr(5) * (V(1) - V(4)));

ddz_wFR = (1 / m(2)) * (F(2)...
    + kt(2) * (zB(2) - D(2))...
    - ks(2) * (D(2) - D(5) + w(1,2) * D(6) - w(2,2) * D(7))...
    + ct(2) * (dzB(2) - V(2))...
    - cs(2) * (V(2) - V(5) + w(1,2) * V(6) - w(2,2) * V(7))...
    - kr(1) * (D(2) - D(1))...
    - kr(4) * (D(2) - D(4))...
    - kr(6) * (D(2) - D(3))...
    - cr(1) * (V(2) - V(1))...
    - cr(4) * (V(2) - V(4))...
    - cr(6) * (V(2) - V(3)));

ddz_wRL = (1 / m(3)) * (F(3)...
    + kt(3) * (zB(3) - D(3))...
    - ks(3) * (D(3) - D(5) + w(1,3) * D(6) - w(2,3) * D(8))...
    + ct(3) * (dzB(3) - V(3))...
    - cs(3) * (V(3) - V(5) + w(1,3) * V(6) - w(2,3) * V(8))...
    + kr(2) * (D(4) - D(3))...
    + kr(3) * (D(1) - D(3))...
    + kr(6) * (D(2) - D(3))...
    + cr(2) * (V(4) - V(3))...
    + cr(3) * (V(1) - V(3))...
    + cr(6) * (V(2) - V(3)));

ddz_wRR = (1 / m(4)) * (F(4)...
    + kt(4) * (zB(4) - D(4))...
    - ks(4) * (D(4) - D(5) + w(1,4) * D(6) - w(2,4) * D(8))...
    + ct(4) * (dzB(4) - V(4))...
    - cs(4) * (V(4) - V(5) + w(1,4) * V(6) - w(2,4) * V(8))...
    - kr(2) * (D(4) - D(3))...
    + kr(4) * (D(2) - D(4))...
    + kr(5) * (D(1) - D(4))...
    - cr(2) * (V(4) - V(3))...
    + cr(4) * (V(2) - V(4))...
    + cr(5) * (V(1) - V(4)));

ddz_c = (1 / m(5)) * (F(5)...
    + ks(1) * (D(1) - D(5) + w(1,1) * D(6) - w(2,1) * D(7))...
    + ks(2) * (D(2) - D(5) + w(1,2) * D(6) - w(2,2) * D(7))...
    + ks(3) * (D(3) - D(5) + w(1,3) * D(6) - w(2,3) * D(8))...
    + ks(4) * (D(4) - D(5) + w(1,4) * D(6) - w(2,4) * D(8))...
    + cs(1) * (V(1) - V(5) + w(1,1) * V(6) - w(2,1) * V(7))...
    + cs(2) * (V(2) - V(5) + w(1,2) * V(6) - w(2,2) * V(7))...
    + cs(3) * (V(3) - V(5) + w(1,3) * V(6) - w(2,3) * V(8))...
    + cs(4) * (V(4) - V(5) + w(1,4) * V(6) - w(2,4) * V(8)));

ddthetay_c = (1 / I(1)) * (F(6)...
    - w(1,1) * ks(1) * (D(1) - D(5) + w(1,1) * D(6) - w(2,1) * D(7))...
    - w(1,2) * ks(2) * (D(2) - D(5) + w(1,2) * D(6) - w(2,2) * D(7))...
    - w(1,3) * ks(3) * (D(3) - D(5) + w(1,3) * D(6) - w(2,3) * D(8))...
    - w(1,4) * ks(4) * (D(4) - D(5) + w(1,4) * D(6) - w(2,4) * D(8))...
    - w(1,1) * cs(1) * (V(1) - V(5) + w(1,1) * V(6) - w(2,1) * V(7))...
    - w(1,2) * cs(2) * (V(2) - V(5) + w(1,2) * V(6) - w(2,2) * V(7))...
    - w(1,3) * cs(3) * (V(3) - V(5) + w(1,3) * V(6) - w(2,3) * V(8))...
    - w(1,4) * cs(4) * (V(4) - V(5) + w(1,4) * V(6) - w(2,4) * V(8)));

dthetax_F = (1 / I(2)) * (F(7)...
    + w(2,1) * ks(1) * (D(1) - D(5) + w(1,1) * D(6) - w(2,1) * D(7))...
    + w(2,2) * ks(2) * (D(2) - D(5) + w(1,2) * D(6) - w(2,2) * D(7))...
    - kc(1) * (D(7) - D(8))...
    + w(2,1) * cs(1) * (V(1) - V(5) + w(1,1) * V(6) - w(2,1) * V(7))...
    + w(2,2) * cs(2) * (V(2) - V(5) + w(1,2) * V(6) - w(2,2) * V(7))...
    - cc(1) * (V(7) - V(8)));

ddthetax_R = (1 / I(3)) * (F(8)...
	+ w(2,3) * ks(3) * (D(3) - D(5) + w(1,3) * D(6) - w(2,3) * D(8))...
    + w(2,4) * ks(4) * (D(4) - D(5) + w(1,4) * D(6) - w(2,4) * D(8))...
    + kc(1) * (D(7) - D(8))...
	+ w(2,3) * cs(3) * (V(3) - V(5) + w(1,3) * V(6) - w(2,3) * V(8))...
    + w(2,4) * cs(4) * (V(4) - V(5) + w(1,4) * V(6) - w(2,4) * V(8))...
    + cc(1) * (D(7) - D(8)));

A = [ddz_wFL;ddz_wFR;ddz_wRL;ddz_wRR;ddz_c;ddthetay_c;dthetax_F;ddthetax_R];

== matlab function EVX_Lap_Simulation/EVX Vehicle Model/Vertical Dynamics/MATLAB Function2 ==
  data: zB output
function zB = fcn()

% Base Displacements

% zB_FL = 0;
% zB_FR = 0;
% zB_RL = 0;
% zB_RR = 0;
% 
% if t > 2
%     zB_FL = 0.01;
%     zB_RL = 0.00;
% end
% 
% if t > 3
%     zB_FL = 0.01;
%     zB_RL = 0.01;
% end
% 
% if t > 4
%     zB_FL = 0.015;
%     zB_RL = 0.015;
% end
% 
% if t > 5
%     zB_FL = 0;
%     zB_RL = 0;
% end
% 
% if t > 7
% zB_FL = 0.001 * sin(2*t);
% zB_FR = -0.001 * sin(2*t);
% zB_RL = 0.001 * sin(2*t);
% zB_RR = -0.001 * sin(2*t);
% end
% 
% if t > 15
% zB_FL = 0.001 * sin(3*t) - 0.005;
% zB_FR = -0.001 * sin(3*t);
% zB_RL = 0.001 * sin(3*t) - 0.005;
% zB_RR = -0.001 * sin(3*t);
% end

zB_FL = 0;
zB_FR = 0;
zB_RL = 0;
zB_RR = 0;

zB = [zB_FL,zB_FR,zB_RL,zB_RR];
